simulink model "elipse"  (R2020b)
settings: Solver=VariableStepAuto  StartTime=0.0  StopTime=1000.0  RelTol=1e-3
libraries: simulink x1
settings Model: Creator=morro  LastModifiedBy=morro

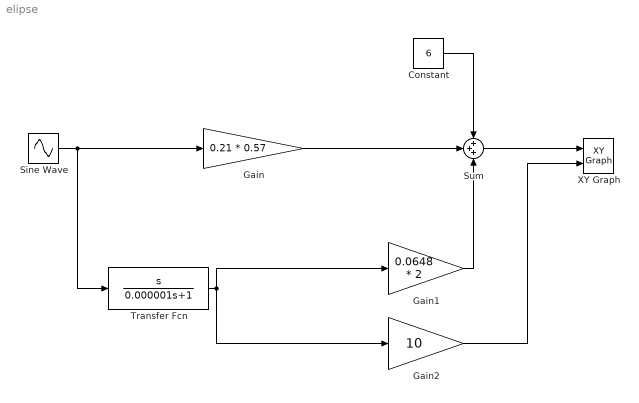
== system elipse ==
  Constant : Constant  Value=6
  Gain : Gain  Gain=0.21 * 0.57
  Gain1 : Gain  Gain=0.0648 * 2
  Gain2 : Gain  Gain=10
  Sine Wave : Sin  Amplitude=3.5  Frequency=0.57  SampleTime=0
  Sum : Sum  Inputs=+++
  Transfer Fcn : TransferFcn  Numerator=[1 0]  Denominator=[0.000001 1]
  XY Graph : simulink/Sinks/XY Graph  xmin=4  xmax=8  ymin=-25  ymax=25  st=-1
  wires:
  Gain2/1 -> XY Graph/2
  Transfer Fcn/1 -> Gain2/1, Gain1/1
  Gain/1 -> Sum/2
  Sine Wave/1 -> Transfer Fcn/1, Gain/1
  Gain1/1 -> Sum/3
  Sum/1 -> XY Graph/1
  Constant/1 -> Sum/1
